simulink model "controlBlockDevelopment_generic_compat"  (Simulink 8.7)
settings: Solver=ode45  StartTime=0.0  StopTime=60  RelTol=1e-3
undefined symbols (not defined in the file): my_joint
libraries: simulink x1, cjt_library_models x1
settings Model: Creator=joern  LastModifiedBy=J�rn
settings DebuggingCC: UnderspecifiedInitializationDetection=Simplified  MergeDetectMultiDrivingBlocksExec=error  SolverPrmCheckMsg=warning  AllowSymbolicDim=off
settings ConfigComp: CovModelRefEnable=off

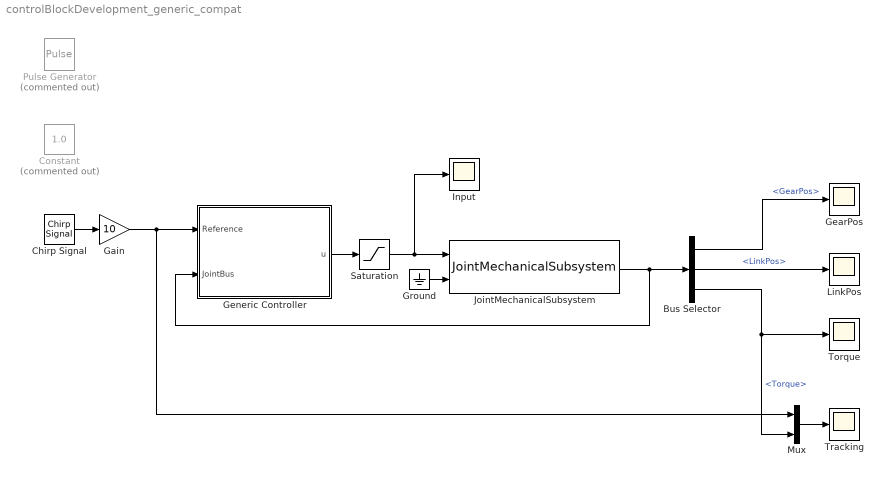
== system controlBlockDevelopment_generic_compat ==
  Bus Selector : BusSelector  OutputSignals=GearPos,LinkPos,Torque
  Chirp Signal : simulink/Sources/Chirp Signal  f1=0.1  T=60  f2=60
  Constant : Constant  Commented=on  Value=1.0
  Gain : Gain  Gain=10
  GearPos : Scope
  Generic Controller : Subsystem  mask{jointObj=my_joint}
      mask prompts: jointObj "Joint Object"
      mask init:
      | % Get linear dynamics matrices
      | [A, B, C, I, D, K] = jointObj.getDynamicsMatrices();
  Ground : Ground
  Input : Scope
  JointMechanicalSubsystem : cjt_library_models/Joint models/JointMechanicalSubsystem  jointObj=jointObj  fc_vel=499  fc_torque=499  input_delay=1  output_delay=1  quantize=on  quantize_bits=19  input_noise_enabled=off  output_noise_enabled=off  var_u=0.12^2  var_y=1.8e-10
  LinkPos : Scope
  Mux : Mux  Inputs=2
  Pulse Generator : DiscretePulseGenerator  Commented=on  PulseType=Time based  Period=10  PulseWidth=0.1
  Saturation : Saturate  UpperLimit=40  LowerLimit=-40
  Torque : Scope
  Tracking : Scope
  wires:
  JointMechanicalSubsystem/1 -> Bus Selector/1, Generic Controller/2(JointBus)
  Bus Selector/2 -> LinkPos/1  "<LinkPos>"
  Bus Selector/3 -> Torque/1, Mux/2  "<Torque>"
  Mux/1 -> Tracking/1
  Bus Selector/1 -> GearPos/1  "<GearPos>"
  Chirp Signal/1 -> Gain/1
  Gain/1 -> Generic Controller/1(Reference), Mux/1
  Generic Controller/1(u) -> Saturation/1
  Saturation/1 -> JointMechanicalSubsystem/1, Input/1
  Ground/1 -> JointMechanicalSubsystem/2

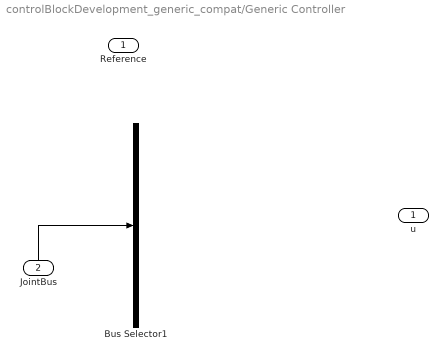
== system controlBlockDevelopment_generic_compat/Generic Controller ==
  Reference : Inport
  JointBus : Inport  Port=2
  Bus Selector1 : BusSelector  OutputSignals=GearPos,LinkPos,Torque
  u : Outport
  wires:
  JointBus/1 -> Bus Selector1/1
